simulink model "ARC_DTm"  (R2025b)
settings: Solver=FixedStepAuto  StartTime=0.0  StopTime=10080  FixedStep=1  RelTol=1e-3
PreLoadFcn:
  | %For Preload, set the working path
  | modelFolder = fileparts(which(bdroot));
  | addpath(genpath(modelFolder));
StartFcn:
  | tic
StopFcn:
  | fprintf("Sim Time: %.02f min", toc/60)
values from neighbouring files (symbols this model uses):
  batteryScenario = p.batteryScenario    [RUNSIM_ParameterSweep.m]    (also in _RUNSIM_ParameterSweep.m)
  Electricity_SalePriceModifier = 50/100    (= 0.5)    [RUNSIM_ParameterSweep.m]    (also in _RUNSIM_ParameterSweep.m)
  LUT = LUT_load.gamLUT    [RUNSIM_ParameterSweep.m]    (also in _RUNSIM_ParameterSweep.m)
  minimum_UF_system_flow = 5833    [RUNSIM_ParameterSweep.m]    (also in _RUNSIM_ParameterSweep.m)
  PROS1_recoveryrate = 61    [RUNSIM_ParameterSweep.m]    (also in _RUNSIM_ParameterSweep.m)
  PROS2_recoveryrate = 62    [RUNSIM_ParameterSweep.m]    (also in _RUNSIM_ParameterSweep.m)
  ROstabilization_time = p.ROstabilization_time    [RUNSIM_ParameterSweep.m]    (also in _RUNSIM_ParameterSweep.m)
  solarModifier = maximum_solar_generation / 300    [RUNSIM_ParameterSweep.m]    (also in _RUNSIM_ParameterSweep.m)
  TSRO_recoveryrate = 51    [RUNSIM_ParameterSweep.m]    (also in _RUNSIM_ParameterSweep.m)
  UF_RecoveryRate = 96    [RUNSIM_ParameterSweep.m]    (also in _RUNSIM_ParameterSweep.m)
undefined symbols (not defined in the file or in its folder): A_PROS1, A_PROS2, A_TSRO, B_PROS1, B_PROS2, B_TSRO, BW_Max_Time, BW_Max_Vol_gal, CEB_Max_Time, CEB_Max_Vol_gal, CIP_Max_Time, E, FF, h, L, w
libraries: simulink x40
(part 8 of 11)

== system ARC_DTm/Plant_LocalLoad_FMU/Battery System/Battery PID Solar Data1 ==
  note: M=2.5, kp=2.965, Ti=166.5, ki=0.0178
      |
      | M=1.5, kp=4.9, Ti=99.9, ki=0.049
      |
      | M=0.5, kp=14.8, Ti=33.3, ki=0.4
      |
      | M=0.1, kp=74.13, Ti=6.66, ki=11.13
      |
      | M=0.055 kp=134.79, Ti=3.663, ki=36.79
      |
      | M=0.01, kp=741.35, Ti=0.666, ki=1112.8
      |
      | M=0.001, kp=7413.5, Ti=0.0666, ki=111,313.81
      |
      | M=0.0001, kp=74135.09, Ti=0.00666, ki=11,113,394.89
  Setpoint : Inport
  feedback : Inport  Port=2
  Add : Sum
  BatteryCharge : Saturate  UpperLimit=0  LowerLimit=-1
  Constant : Constant  Value=0
  Dead Zone : DeadZone  LowerValue=-0.01  UpperValue=0.01
  Dead Zone1 : DeadZone  LowerValue=-0.025  UpperValue=0.025
  Gain7 : Gain  Gain=134.79
  Gain8 : Gain  Gain=36.79
  Manual Switch : ManualSwitch
  Proportional3 : Gain  SaturateOnIntegerOverflow=on  OutDataTypeStr=Inherit: Same as input  ParamDataTypeStr=Inherit: Same as input
  Scope : Scope  NumInputPorts=3
      settings: ActiveDisplayYMinimum=-113.50359317586926  ActiveDisplayYMaximum=90.190900765776917  DataLoggingVariableName=ScopeData4
  Scope1 : Scope
      settings: ActiveDisplayYMinimum=-1  ActiveDisplayYMaximum=1  DataLoggingVariableName=ScopeData8
  Scope2 : Scope  NumInputPorts=4
      settings: Title=Setpoint  ActiveDisplayYMinimum=-0.96522618550308326  ActiveDisplayYMaximum=1.0322332098634432  DataLoggingVariableName=ScopeData2
  Subtract : Sum  Inputs=+-
  Subtract1 : Sum  Inputs=+-
  Sum1 : Sum  Inputs=|+-
  Sum6 : Sum  Inputs=+-  InputSameDT=on  SaturateOnIntegerOverflow=on  OutDataTypeStr=Inherit: Same as first input
  Unit Delay : UnitDelay  SampleTime=-1  HasFrameUpgradeWarning=on
  Unit Delay1 : UnitDelay  SampleTime=-1  HasFrameUpgradeWarning=on
  open-loop steps : Subsystem
  Battery Disch : Outport
  wires:
  Manual Switch/1 -> Battery Disch/1
  open-loop steps/1(Out1) -> Manual Switch/2
  Setpoint/1 -> Scope2/1, Subtract1/1
  Proportional3/1 -> Subtract/2
  feedback/1 -> Scope2/2, Subtract1/2
  Sum1/1 -> Add/2, Unit Delay/1
  Subtract/1 -> Scope1/1, Sum1/1
  Unit Delay/1 -> Sum1/2
  Subtract1/1 -> Gain8/1, Gain7/1, Scope2/3
  BatteryCharge/1 -> Sum6/2, Scope2/4, Manual Switch/1, Scope/2
  Add/1 -> Scope/1, BatteryCharge/1, Sum6/1
  Gain7/1 -> Add/1
  Gain8/1 -> Subtract/1
  Sum6/1 -> Proportional3/1, Scope/3

== system ARC_DTm/Plant_LocalLoad_FMU/Battery System/Battery PID Solar Data2 ==
  note: M=2.5, kp=2.965, Ti=166.5, ki=0.0178
      |
      | M=1.5, kp=4.9, Ti=99.9, ki=0.049
      |
      | M=0.5, kp=14.8, Ti=33.3, ki=0.4
      |
      | M=0.1, kp=74.13, Ti=6.66, ki=11.13
      |
      | M=0.055 kp=134.79, Ti=3.663, ki=36.79
      |
      | M=0.01, kp=741.35, Ti=0.666, ki=1112.8
      |
      | M=0.001, kp=7413.5, Ti=0.0666, ki=111,313.81
      |
      | M=0.0001, kp=74135.09, Ti=0.00666, ki=11,113,394.89
  Setpoint : Inport
  feedback : Inport  Port=2
  Add : Sum
  BatteryCharge : Saturate  UpperLimit=1  LowerLimit=0
  Constant : Constant  Value=0
  Dead Zone : DeadZone  LowerValue=-0.01  UpperValue=0.01
  Dead Zone1 : DeadZone  LowerValue=-0.025  UpperValue=0.025
  Gain7 : Gain  Gain=134.79
  Gain8 : Gain  Gain=36.79
  Manual Switch : ManualSwitch
  Proportional3 : Gain  SaturateOnIntegerOverflow=on  OutDataTypeStr=Inherit: Same as input  ParamDataTypeStr=Inherit: Same as input
  Scope : Scope  NumInputPorts=3
      settings: ActiveDisplayYMinimum=-39.201768628012239  ActiveDisplayYMaximum=109.61089187015484  DataLoggingVariableName=ScopeData4
  Scope1 : Scope
      settings: ActiveDisplayYMinimum=-1  ActiveDisplayYMaximum=1  DataLoggingVariableName=ScopeData9
  Scope2 : Scope  NumInputPorts=4
      settings: Title=Setpoint  ActiveDisplayYMinimum=-0.96522618502196855  ActiveDisplayYMaximum=1.0322332055334107  DataLoggingVariableName=ScopeData2
  Scope3 : Scope  NumInputPorts=2
      settings: ActiveDisplayYMinimum=-0.25471317003362626  ActiveDisplayYMaximum=0.79251853030263664  DataLoggingVariableName=ScopeData2
  Subtract : Sum  Inputs=+-
  Subtract1 : Sum  Inputs=+-
  Sum1 : Sum  Inputs=|+-
  Sum6 : Sum  Inputs=+-  InputSameDT=on  SaturateOnIntegerOverflow=on  OutDataTypeStr=Inherit: Same as first input
  Unit Delay : UnitDelay  SampleTime=-1  HasFrameUpgradeWarning=on
  open-loop steps : Subsystem
  BatteryChargeDisch : Outport
  wires:
  Manual Switch/1 -> BatteryChargeDisch/1
  open-loop steps/1(Out1) -> Manual Switch/2
  Setpoint/1 -> Scope2/1, Subtract1/1
  Proportional3/1 -> Subtract/2
  feedback/1 -> Scope2/2, Subtract1/2
  Sum1/1 -> Add/2, Unit Delay/1
  Subtract/1 -> Scope1/1, Sum1/1
  Unit Delay/1 -> Sum1/2
  Subtract1/1 -> Scope3/2, Gain8/1, Gain7/1, Scope2/3, Scope3/1
  BatteryCharge/1 -> Scope2/4, Manual Switch/1, Sum6/2, Scope/2
  Add/1 -> Scope/1, Sum6/1, BatteryCharge/1
  Gain7/1 -> Add/1
  Gain8/1 -> Subtract/1
  Sum6/1 -> Proportional3/1, Scope/3

== system ARC_DTm/Plant_LocalLoad_FMU/Battery System/Battery PID Solar Data3 ==
  note: M=2.5, kp=2.965, Ti=166.5, ki=0.0178
      |
      | M=1.5, kp=4.9, Ti=99.9, ki=0.049
      |
      | M=0.5, kp=14.8, Ti=33.3, ki=0.4
      |
      | M=0.1, kp=74.13, Ti=6.66, ki=11.13
      |
      | M=0.055 kp=134.79, Ti=3.663, ki=36.79
      |
      | M=0.01, kp=741.35, Ti=0.666, ki=1112.8
      |
      | M=0.001, kp=7413.5, Ti=0.0666, ki=111,313.81
      |
      | M=0.0001, kp=74135.09, Ti=0.00666, ki=11,113,394.89
  Setpoint : Inport
  feedback : Inport  Port=2
  Add : Sum
  BatteryCharge : Saturate  UpperLimit=0  LowerLimit=-1
  Constant : Constant  Value=0
  Dead Zone : DeadZone  LowerValue=-0.01  UpperValue=0.01
  Dead Zone1 : DeadZone  LowerValue=-0.025  UpperValue=0.025
  Gain7 : Gain  Gain=134.79
  Gain8 : Gain  Gain=36.79
  Manual Switch : ManualSwitch
  Proportional3 : Gain  SaturateOnIntegerOverflow=on  OutDataTypeStr=Inherit: Same as input  ParamDataTypeStr=Inherit: Same as input
  Scope : Scope  NumInputPorts=3
      settings: ActiveDisplayYMinimum=-113.50359317586926  ActiveDisplayYMaximum=90.190900765776917  DataLoggingVariableName=ScopeData4
  Scope1 : Scope
      settings: ActiveDisplayYMinimum=-1  ActiveDisplayYMaximum=1  DataLoggingVariableName=ScopeData8
  Scope2 : Scope  NumInputPorts=4
      settings: Title=Setpoint  ActiveDisplayYMinimum=-0.96522618550308326  ActiveDisplayYMaximum=1.0322332098634432  DataLoggingVariableName=ScopeData2
  Subtract : Sum  Inputs=+-
  Subtract1 : Sum  Inputs=+-
  Sum1 : Sum  Inputs=|+-
  Sum6 : Sum  Inputs=+-  InputSameDT=on  SaturateOnIntegerOverflow=on  OutDataTypeStr=Inherit: Same as first input
  Unit Delay : UnitDelay  SampleTime=-1  HasFrameUpgradeWarning=on
  Unit Delay1 : UnitDelay  SampleTime=-1  HasFrameUpgradeWarning=on
  open-loop steps : Subsystem
  Battery Disch : Outport
  wires:
  Manual Switch/1 -> Battery Disch/1
  open-loop steps/1(Out1) -> Manual Switch/2
  Setpoint/1 -> Scope2/1, Subtract1/1
  Proportional3/1 -> Subtract/2
  feedback/1 -> Scope2/2, Subtract1/2
  Sum1/1 -> Add/2, Unit Delay/1
  Subtract/1 -> Scope1/1, Sum1/1
  Unit Delay/1 -> Sum1/2
  Subtract1/1 -> Gain8/1, Gain7/1, Scope2/3
  BatteryCharge/1 -> Sum6/2, Scope2/4, Manual Switch/1, Scope/2
  Add/1 -> Scope/1, BatteryCharge/1, Sum6/1
  Gain7/1 -> Add/1
  Gain8/1 -> Subtract/1
  Sum6/1 -> Proportional3/1, Scope/3

== system ARC_DTm/Plant_LocalLoad_FMU/Battery System/Excess Solar ==
  Solar In : Inport
  Local Load Demand : Inport  Port=2
  Action Port : ActionPort  ActionPortLabel=if(u1 == 1)
  Battery PID Solar Data : Subsystem  Commented=on
  Battery PID Solar Data1 : Subsystem  Commented=on
  Cast To Double : DataTypeConversion  OutDataTypeStr=double  SaturateOnIntegerOverflow=off  RndMeth=Floor
  Cast To Double1 : DataTypeConversion  OutDataTypeStr=double  SaturateOnIntegerOverflow=off  RndMeth=Floor
  Compare To Zero : simulink/Logic and Bit Operations/Compare To Zero  relop=>=  OutDataTypeStr=boolean
  Compare To Zero1 : simulink/Logic and Bit Operations/Compare To Zero  relop=<  OutDataTypeStr=boolean
  From1 : From  Commented=on  GotoTag=SOC
  From2 : From  Commented=on  GotoTag=SOC
  Gain : Gain  Commented=on  Gain=-1
  Goto : Goto  Commented=on  GotoTag=SOC
  Scope : Scope  Commented=on  NumInputPorts=2
      settings: ActiveDisplayYMinimum=-1.0125  ActiveDisplayYMaximum=0.11249999999999998  DataLoggingVariableName=ScopeData27
  Scope1 : Scope  Commented=on  NumInputPorts=2
      settings: ActiveDisplayYMinimum=-0.96522618502196855  ActiveDisplayYMaximum=1.0322332055334107  DataLoggingVariableName=ScopeData37
  "Setpoint PID Solar+Battery " : Subsystem  Commented=on
  Sum : Sum  Inputs=|+-
  Unit Delay1 : UnitDelay  Commented=on  SampleTime=-1  HasFrameUpgradeWarning=on
  Unit Delay2 : UnitDelay  Commented=on  SampleTime=-1  HasFrameUpgradeWarning=on
  Battery Charge Command : Outport
  Battery Discharge Command : Outport  Port=2
  wires:
  Gain/1 -> Scope/2
  Unit Delay2/1 -> Battery PID Solar Data1/2(feedback)
  "Setpoint PID Solar+Battery "/2(Setpoint BattDischarge) -> Scope/1, Battery PID Solar Data1/1(Setpoint)
  "Setpoint PID Solar+Battery "/1(Setpoint BattCharge) -> Scope1/1, Battery PID Solar Data/1(Setpoint)
  From1/1 -> Unit Delay1/1
  Battery PID Solar Data1/1(Battery Disch) -> Gain/1
  From2/1 -> Unit Delay2/1
  Unit Delay1/1 -> Battery PID Solar Data/2(feedback)
  Battery PID Solar Data/1(BatteryChargeDisch) -> Scope1/2
  Solar In/1 -> Sum/1
  Local Load Demand/1 -> Sum/2
  Sum/1 -> Compare To Zero1/1, Compare To Zero/1
  Compare To Zero/1 -> Cast To Double1/1
  Compare To Zero1/1 -> Cast To Double/1
  Cast To Double/1 -> Battery Discharge Command/1
  Cast To Double1/1 -> Battery Charge Command/1

== system ARC_DTm/Plant_LocalLoad_FMU/Battery System/NoBattery ==
  Action Port : ActionPort  ActionPortLabel=else
  No Charge : Constant  Value=0
  Battery Charge Request : Outport
  Battery Discharge Request : Outport  Port=2
  wires:
  No Charge/1 -> Battery Discharge Request/1, Battery Charge Request/1

== system ARC_DTm/Plant_LocalLoad_FMU/Battery System/Setpoint PID Solar+Battery  ==
  Solar Power : Inport
  Local Load Demand : Inport  Port=2
  Divide : Product  Inputs=*/
  Rate Limiter1 : RateLimiter  RisingSlewLimit=0.00000607  FallingSlewLimit=-0.00000607  SampleTimeMode=inherited
  Rate Limiter2 : RateLimiter  RisingSlewLimit=0.00000607  FallingSlewLimit=-0.00000607  SampleTimeMode=inherited
  Saturation1 : Saturate  UpperLimit=0.9  LowerLimit=-0.9
  Saturation4 : Saturate  UpperLimit=0.9  LowerLimit=-0.9
  Scaling factor Solar Data to 1 MW Battery : Constant  Value=10000
  Scope7 : Scope  NumInputPorts=3
      settings: Title=Battery Charge/Discharge SOC Output  ActiveDisplayYMinimum=-0.95011803109224124  ActiveDisplayYMaximum=0.10556867012136011
  Subtract2 : Sum  Inputs=+-
  Transfer Fcn3 : TransferFcn  Denominator=[300 1]
  Setpoint BattCharge : Outport
  Setpoint BattDischarge : Outport  Port=2
  wires:
  Subtract2/1 -> Scope7/1, Transfer Fcn3/1
  Transfer Fcn3/1 -> Divide/1
  Local Load Demand/1 -> Subtract2/2
  Solar Power/1 -> Subtract2/1
  Divide/1 -> Saturation1/1, Saturation4/1
  Saturation4/1 -> Setpoint BattCharge/1, Scope7/2
  Saturation1/1 -> Scope7/3, Setpoint BattDischarge/1
  Scaling factor Solar Data to 1 MW Battery/1 -> Divide/2

== system ARC_DTm/Product Water Tank/Tank Storage/Manage Overflows ==
  Timer : Inport
  <Flow Rate (FLOW)> : Inport  Port=2
  <Permeate Flow (FLOW)> : Inport  Port=3
  Pump Flow (FLOW) : Inport  Port=4
  If : If  IfExpression=u1 >= 1  ElseIfExpressions=u1<= -1
  If Action Subsystem : Subsystem  TreatAsAtomicUnit=on
  If Action Subsystem1 : Subsystem  TreatAsAtomicUnit=on
  Merge : Merge  Inputs=3
  Merge1 : Merge  Inputs=3
  Merge2 : Merge  Inputs=3
  Pump Flow Reduction : Subsystem  TreatAsAtomicUnit=on
  Reduce to Zero : MATLAB Function  TreatAsAtomicUnit=on
  Scope : Scope
      settings: ActiveDisplayYMinimum=-18.75  ActiveDisplayYMaximum=18.75  DataLoggingVariableName=ScopeData2
  Well Flow Rate (FLOW) : Outport
  RO Perm Flow Rate (FLOW) : Outport  Port=2
  Pump Flow Rate (FLOW) : Outport  Port=3
  TimerOut : Outport  Port=4
  wires:
  Timer/1 -> Reduce to Zero/1(u), Scope/1, If/1
  If/1 -> If Action Subsystem/Action
  <Flow Rate (FLOW)>/1 -> Pump Flow Reduction/1(<Flow Rate (FLOW)>), If Action Subsystem/1(<Flow Rate (FLOW)>), If Action Subsystem1/1(<Flow Rate (FLOW)>)
  <Permeate Flow (FLOW)>/1 -> Pump Flow Reduction/2(<PermeateFlow (FLOW)>), If Action Subsystem/2(<Permeate Flow (FLOW)>), If Action Subsystem1/2(<Permeate Flow (FLOW)>)
  Pump Flow (FLOW)/1 -> If Action Subsystem/3(Pump Flow (FLOW)), If Action Subsystem1/3(<Pump Flow (FLOW)>)
  If Action Subsystem/1(Raw Water Flow Rate (FLOW)) -> Merge/1
  If/3 -> If Action Subsystem1/Action
  If Action Subsystem1/1(Well Flow Rate (FLOW)) -> Merge/2
  Merge/1 -> Well Flow Rate (FLOW)/1
  If Action Subsystem/2(RO Permeate Flow Rate (FLOW)) -> Merge1/1
  If Action Subsystem1/2(RO Perm Flow Rate (FLOW)) -> Merge1/2
  Merge1/1 -> RO Perm Flow Rate (FLOW)/1
  Pump Flow Reduction/3(Pump Flow (FLOW)) -> Merge2/3
  Merge2/1 -> Pump Flow Rate (FLOW)/1
  If/2 -> Pump Flow Reduction/Action
  If Action Subsystem1/3(Pump Flow (FLOW)) -> Merge2/2
  If Action Subsystem/3(Pump Flow Rate (FLOW)) -> Merge2/1
  Pump Flow Reduction/2(Permeate Flow Rate (FLOW)) -> Merge1/3
  Pump Flow Reduction/1(Well Flow Rate (FLOW)) -> Merge/3
  Reduce to Zero/1(y) -> TimerOut/1

== system ARC_DTm/Product Water Tank/Tank Storage/VolumeConditions ==
  note: Volume Overflow
  Stored Volume (VOL) : Inport
  Tank Volume (VOL) : Inport  Port=2
  Timer : Inport  Port=3
  If : If  NumInputs=3  IfExpression=u1 >= u2  ElseIfExpressions=u1 <= u3, u3 < u1 < u2  ShowElse=off
  MaximumOperationalVolume : Gain  Gain=volMax
  Merge : Merge  Inputs=3
  MinimumOperationalVolume : Gain  Gain=volMin
  Scope : Scope
      settings: ActiveDisplayYMinimum=-1  ActiveDisplayYMaximum=1  DataLoggingVariableName=ScopeData3
  Tank Above Operating Range : Subsystem  TreatAsAtomicUnit=on
  Tank Below Operating Range : Subsystem  TreatAsAtomicUnit=on
  Tank in Operating Range : Subsystem  TreatAsAtomicUnit=on
  Cooldown Timer : Outport
  wires:
  Tank in Operating Range/1(y) -> Merge/2
  Stored Volume (VOL)/1 -> If/1
  If/1 -> Tank Above Operating Range/Action
  Tank Above Operating Range/1(Out1) -> Merge/1
  Merge/1 -> Scope/1, Cooldown Timer/1
  If/2 -> Tank in Operating Range/Action
  If/3 -> Tank Below Operating Range/Action
  Tank Below Operating Range/1(Out1) -> Merge/3
  Tank Volume (VOL)/1 -> MinimumOperationalVolume/1, MaximumOperationalVolume/1
  MaximumOperationalVolume/1 -> If/2
  MinimumOperationalVolume/1 -> If/3
  Timer/1 -> Tank in Operating Range/1(Timer)

== system ARC_DTm/UF Maintenance Coordinator/arhive/UF_Operation State_1 ==
  UF1_MaintenanceStartSignal : Inport
  UF1_BeginStandby : Inport  Port=2
  UF1_BeginStartup : Inport  Port=3
  Bus Creator : BusCreator  Inputs=2
  Bus Selector : BusSelector  OutputSignals=UF_ShutdownCmd_1
  Bus Selector1 : BusSelector  OutputSignals=UF_MaintCmd_1
  Bus Selector2 : BusSelector  OutputSignals=UF_StartupCmd_1
  Delay Reset Signal : Memory
  Delay Startup : Memory
  UF1_Maintenance State : Stateflow chart  TreatAsAtomicUnit=on
  tag scope: UF1_MaintenanceRequest=global, UF1_MaintenanceState=global, UF1_OperatingState=global, UF1_StartupRequest=global
  wires:
  UF1_Maintenance State/1(unit_in_maint_queue) -> [UF1_MaintenanceRequest]  "UF1_MaintenanceRequestQueue"
  Bus Creator/1 -> [UF1_MaintenanceState]
  Delay Startup/1 -> [UF1_OperatingState], Bus Creator/1  "UF1_OperationsState"
  UF1_Maintenance State/4(maintenance_completion_indicator) -> Delay Reset Signal/1  "UF1_MaintenanceCompletionSignal"
  [UF1_Maintenance_Request] -> UF1_Maintenance State/2(maint_req)
  Delay Reset Signal/1 -> Bus Creator/2  "UF1_MaintenanceCompletionSignal"
  UF1_Maintenance State/3(unit_in_operation) -> Delay Startup/1  "UF1_OperationsState"
  UF1_Maintenance State/2(unit_in_startup_queue) -> [UF1_StartupRequest]  "UF1_StartupRequestQueue"
  UF1_BeginStandby/1 -> Bus Selector/1  "UF1_BeginStandby"
  Bus Selector/1 -> UF1_Maintenance State/3(standby_cmd)  "<UF_ShutdownCmd_1>"
  UF1_MaintenanceStartSignal/1 -> Bus Selector1/1  "UF1_MaintenanceStartSignal"
  Bus Selector1/1 -> UF1_Maintenance State/1(maint_cmd)  "<UF_MaintCmd_1>"
  UF1_BeginStartup/1 -> Bus Selector2/1  "UF1_BeginStartup"
  Bus Selector2/1 -> UF1_Maintenance State/4(startup_cmd)  "<UF_StartupCmd_1>"

== system ARC_DTm/UF Maintenance Coordinator/arhive/UF_Operation State_10 ==
  UF10_MaintenanceStartSignal : Inport
  UF10_BeginStandby : Inport  Port=2
  UF10_BeginStartup : Inport  Port=3
  Bus Creator : BusCreator  Inputs=2
  Bus Selector : BusSelector  OutputSignals=UF_ShutdownCmd_10
  Bus Selector10 : BusSelector  OutputSignals=UF_MaintCmd_10
  Bus Selector2 : BusSelector  OutputSignals=UF_StartupCmd_10
  Delay Reset Signal : Memory
  Delay Startup : Memory
  UF10_Maintenance State : Stateflow chart  TreatAsAtomicUnit=on
  tag scope: UF10_MaintenanceRequest=global, UF10_MaintenanceState=global, UF10_OperatingState=global, UF10_StartupRequest=global
  wires:
  UF10_Maintenance State/1(unit_in_maint_queue) -> [UF10_MaintenanceRequest]  "UF10_MaintenanceRequestQueue"
  Bus Creator/1 -> [UF10_MaintenanceState]
  Delay Startup/1 -> [UF10_OperatingState], Bus Creator/1  "UF10_OperationsState"
  UF10_Maintenance State/4(maintenance_completion_indicator) -> Delay Reset Signal/1  "UF10_MaintenanceCompletionSignal"
  [UF10_Maintenance_Request] -> UF10_Maintenance State/2(maint_req)
  Delay Reset Signal/1 -> Bus Creator/2  "UF10_MaintenanceCompletionSignal"
  UF10_Maintenance State/3(unit_in_operation) -> Delay Startup/1  "UF10_OperationsState"
  UF10_Maintenance State/2(unit_in_startup_queue) -> [UF10_StartupRequest]  "UF10_StartupRequestQueue"
  UF10_BeginStandby/1 -> Bus Selector/1  "UF10_BeginStandby"
  Bus Selector/1 -> UF10_Maintenance State/3(standby_cmd)  "<UF_ShutdownCmd_10>"
  UF10_MaintenanceStartSignal/1 -> Bus Selector10/1  "UF10_MaintenanceStartSignal"
  Bus Selector10/1 -> UF10_Maintenance State/1(maint_cmd)  "<UF_MaintCmd_10>"
  UF10_BeginStartup/1 -> Bus Selector2/1  "UF10_BeginStartup"
  Bus Selector2/1 -> UF10_Maintenance State/4(startup_cmd)  "<UF_StartupCmd_10>"

== system ARC_DTm/UF Maintenance Coordinator/arhive/UF_Operation State_2 ==
  UF2_MaintenanceStartSignal : Inport
  UF2_BeginStandby : Inport  Port=2
  UF2_BeginStartup : Inport  Port=3
  Bus Creator : BusCreator  Inputs=2
  Bus Selector : BusSelector  OutputSignals=UF_ShutdownCmd_2
  Bus Selector1 : BusSelector  OutputSignals=UF_MaintCmd_2
  Bus Selector2 : BusSelector  OutputSignals=UF_StartupCmd_2
  Delay Reset Signal : Memory
  Delay Startup : Memory
  UF2_Maintenance State : Stateflow chart  TreatAsAtomicUnit=on
  tag scope: UF2_MaintenanceRequest=global, UF2_MaintenanceState=global, UF2_OperatingState=global, UF2_StartupRequest=global
  wires:
  UF2_Maintenance State/1(unit_in_maint_queue) -> [UF2_MaintenanceRequest]  "UF2_MaintenanceRequestQueue"
  Bus Creator/1 -> [UF2_MaintenanceState]
  UF2_Maintenance State/4(maintenance_completion_indicator) -> Delay Reset Signal/1  "UF2_MaintenanceCompletionSignal"
  [UF2_Maintenance_Request] -> UF2_Maintenance State/2(maint_req)
  Delay Reset Signal/1 -> Bus Creator/2  "UF2_MaintenanceCompletionSignal"
  UF2_Maintenance State/3(unit_in_operation) -> Delay Startup/1  "UF2_OperationsState"
  UF2_Maintenance State/2(unit_in_startup_queue) -> [UF2_StartupRequest]  "UF2_StartupRequestQueue"
  UF2_BeginStandby/1 -> Bus Selector/1  "UF2_BeginStandby"
  Bus Selector/1 -> UF2_Maintenance State/3(standby_cmd)  "<UF_ShutdownCmd_2>"
  UF2_MaintenanceStartSignal/1 -> Bus Selector1/1  "UF2_MaintenanceStartSignal"
  Bus Selector1/1 -> UF2_Maintenance State/1(maint_cmd)  "<UF_MaintCmd_2>"
  UF2_BeginStartup/1 -> Bus Selector2/1  "UF2_BeginStartup"
  Bus Selector2/1 -> UF2_Maintenance State/4(startup_cmd)  "<UF_StartupCmd_2>"
  Delay Startup/1 -> [UF2_OperatingState], Bus Creator/1  "UF2_OperationsState"

== system ARC_DTm/UF Maintenance Coordinator/arhive/UF_Operation State_3 ==
  UF3_MaintenanceStartSignal : Inport
  UF3_BeginStandby : Inport  Port=2
  UF3_BeginStartup : Inport  Port=3
  Bus Creator : BusCreator  Inputs=2
  Bus Selector : BusSelector  OutputSignals=UF_ShutdownCmd_3
  Bus Selector2 : BusSelector  OutputSignals=UF_StartupCmd_3
  Bus Selector3 : BusSelector  OutputSignals=UF_MaintCmd_3
  Delay Reset Signal : Memory
  Delay Startup : Memory
  UF3_Maintenance State : Stateflow chart  TreatAsAtomicUnit=on
  tag scope: UF3_MaintenanceRequest=global, UF3_MaintenanceState=global, UF3_OperatingState=global, UF3_StartupRequest=global
  wires:
  UF3_Maintenance State/1(unit_in_maint_queue) -> [UF3_MaintenanceRequest]  "UF3_MaintenanceRequestQueue"
  Bus Creator/1 -> [UF3_MaintenanceState]
  Delay Startup/1 -> [UF3_OperatingState], Bus Creator/1  "UF3_OperationsState"
  UF3_Maintenance State/4(maintenance_completion_indicator) -> Delay Reset Signal/1  "UF3_MaintenanceCompletionSignal"
  [UF3_Maintenance_Request] -> UF3_Maintenance State/2(maint_req)
  Delay Reset Signal/1 -> Bus Creator/2  "UF3_MaintenanceCompletionSignal"
  UF3_Maintenance State/3(unit_in_operation) -> Delay Startup/1  "UF3_OperationsState"
  UF3_Maintenance State/2(unit_in_startup_queue) -> [UF3_StartupRequest]  "UF3_StartupRequestQueue"
  UF3_BeginStandby/1 -> Bus Selector/1  "UF3_BeginStandby"
  Bus Selector/1 -> UF3_Maintenance State/3(standby_cmd)  "<UF_ShutdownCmd_3>"
  UF3_MaintenanceStartSignal/1 -> Bus Selector3/1  "UF3_MaintenanceStartSignal"
  Bus Selector3/1 -> UF3_Maintenance State/1(maint_cmd)  "<UF_MaintCmd_3>"
  UF3_BeginStartup/1 -> Bus Selector2/1  "UF3_BeginStartup"
  Bus Selector2/1 -> UF3_Maintenance State/4(startup_cmd)  "<UF_StartupCmd_3>"

== system ARC_DTm/UF Maintenance Coordinator/arhive/UF_Operation State_4 ==
  UF4_MaintenanceStartSignal : Inport
  UF4_BeginStandby : Inport  Port=2
  UF4_BeginStartup : Inport  Port=3
  Bus Creator : BusCreator  Inputs=2
  Bus Selector : BusSelector  OutputSignals=UF_ShutdownCmd_4
  Bus Selector2 : BusSelector  OutputSignals=UF_StartupCmd_4
  Bus Selector4 : BusSelector  OutputSignals=UF_MaintCmd_4
  Delay Reset Signal : Memory
  Delay Startup : Memory
  UF4_Maintenance State : Stateflow chart  TreatAsAtomicUnit=on
  tag scope: UF4_MaintenanceRequest=global, UF4_MaintenanceState=global, UF4_OperatingState=global, UF4_StartupRequest=global
  wires:
  UF4_Maintenance State/1(unit_in_maint_queue) -> [UF4_MaintenanceRequest]  "UF4_MaintenanceRequestQueue"
  Bus Creator/1 -> [UF4_MaintenanceState]
  Delay Startup/1 -> [UF4_OperatingState], Bus Creator/1  "UF4_OperationsState"
  UF4_Maintenance State/4(maintenance_completion_indicator) -> Delay Reset Signal/1  "UF4_MaintenanceCompletionSignal"
  [UF4_Maintenance_Request] -> UF4_Maintenance State/2(maint_req)
  Delay Reset Signal/1 -> Bus Creator/2  "UF4_MaintenanceCompletionSignal"
  UF4_Maintenance State/3(unit_in_operation) -> Delay Startup/1  "UF4_OperationsState"
  UF4_Maintenance State/2(unit_in_startup_queue) -> [UF4_StartupRequest]  "UF4_StartupRequestQueue"
  UF4_BeginStandby/1 -> Bus Selector/1  "UF4_BeginStandby"
  Bus Selector/1 -> UF4_Maintenance State/3(standby_cmd)  "<UF_ShutdownCmd_4>"
  UF4_MaintenanceStartSignal/1 -> Bus Selector4/1  "UF4_MaintenanceStartSignal"
  Bus Selector4/1 -> UF4_Maintenance State/1(maint_cmd)  "<UF_MaintCmd_4>"
  UF4_BeginStartup/1 -> Bus Selector2/1  "UF4_BeginStartup"
  Bus Selector2/1 -> UF4_Maintenance State/4(startup_cmd)  "<UF_StartupCmd_4>"

== system ARC_DTm/UF Maintenance Coordinator/arhive/UF_Operation State_5 ==
  UF5_MaintenanceStartSignal : Inport
  UF5_BeginStandby : Inport  Port=2
  UF5_BeginStartup : Inport  Port=3
  Bus Creator : BusCreator  Inputs=2
  Bus Selector : BusSelector  OutputSignals=UF_ShutdownCmd_5
  Bus Selector2 : BusSelector  OutputSignals=UF_StartupCmd_5
  Bus Selector5 : BusSelector  OutputSignals=UF_MaintCmd_5
  Delay Reset Signal : Memory
  Delay Startup : Memory
  UF5_Maintenance State : Stateflow chart  TreatAsAtomicUnit=on
  tag scope: UF5_MaintenanceRequest=global, UF5_MaintenanceState=global, UF5_OperatingState=global, UF5_StartupRequest=global
  wires:
  UF5_Maintenance State/1(unit_in_maint_queue) -> [UF5_MaintenanceRequest]  "UF5_MaintenanceRequestQueue"
  Bus Creator/1 -> [UF5_MaintenanceState]
  Delay Startup/1 -> [UF5_OperatingState], Bus Creator/1  "UF5_OperationsState"
  UF5_Maintenance State/4(maintenance_completion_indicator) -> Delay Reset Signal/1  "UF5_MaintenanceCompletionSignal"
  [UF5_Maintenance_Request] -> UF5_Maintenance State/2(maint_req)
  Delay Reset Signal/1 -> Bus Creator/2  "UF5_MaintenanceCompletionSignal"
  UF5_Maintenance State/3(unit_in_operation) -> Delay Startup/1  "UF5_OperationsState"
  UF5_Maintenance State/2(unit_in_startup_queue) -> [UF5_StartupRequest]  "UF5_StartupRequestQueue"
  UF5_BeginStandby/1 -> Bus Selector/1  "UF5_BeginStandby"
  Bus Selector/1 -> UF5_Maintenance State/3(standby_cmd)  "<UF_ShutdownCmd_5>"
  UF5_MaintenanceStartSignal/1 -> Bus Selector5/1  "UF5_MaintenanceStartSignal"
  Bus Selector5/1 -> UF5_Maintenance State/1(maint_cmd)  "<UF_MaintCmd_5>"
  UF5_BeginStartup/1 -> Bus Selector2/1  "UF5_BeginStartup"
  Bus Selector2/1 -> UF5_Maintenance State/4(startup_cmd)  "<UF_StartupCmd_5>"

== system ARC_DTm/UF Maintenance Coordinator/arhive/UF_Operation State_6 ==
  UF6_MaintenanceStartSignal : Inport
  UF6_BeginStandby : Inport  Port=2
  UF6_BeginStartup : Inport  Port=3
  Bus Creator : BusCreator  Inputs=2
  Bus Selector : BusSelector  OutputSignals=UF_ShutdownCmd_6
  Bus Selector2 : BusSelector  OutputSignals=UF_StartupCmd_6
  Bus Selector6 : BusSelector  OutputSignals=UF_MaintCmd_6
  Delay Reset Signal : Memory
  Delay Startup : Memory
  UF6_Maintenance State : Stateflow chart  TreatAsAtomicUnit=on
  tag scope: UF6_MaintenanceRequest=global, UF6_MaintenanceState=global, UF6_OperatingState=global, UF6_StartupRequest=global
  wires:
  UF6_Maintenance State/1(unit_in_maint_queue) -> [UF6_MaintenanceRequest]  "UF6_MaintenanceRequestQueue"
  Bus Creator/1 -> [UF6_MaintenanceState]
  Delay Startup/1 -> [UF6_OperatingState], Bus Creator/1  "UF6_OperationsState"
  UF6_Maintenance State/4(maintenance_completion_indicator) -> Delay Reset Signal/1  "UF6_MaintenanceCompletionSignal"
  [UF6_Maintenance_Request] -> UF6_Maintenance State/2(maint_req)
  Delay Reset Signal/1 -> Bus Creator/2  "UF6_MaintenanceCompletionSignal"
  UF6_Maintenance State/3(unit_in_operation) -> Delay Startup/1  "UF6_OperationsState"
  UF6_Maintenance State/2(unit_in_startup_queue) -> [UF6_StartupRequest]  "UF6_StartupRequestQueue"
  UF6_BeginStandby/1 -> Bus Selector/1  "UF6_BeginStandby"
  Bus Selector/1 -> UF6_Maintenance State/3(standby_cmd)  "<UF_ShutdownCmd_6>"
  UF6_MaintenanceStartSignal/1 -> Bus Selector6/1  "UF6_MaintenanceStartSignal"
  Bus Selector6/1 -> UF6_Maintenance State/1(maint_cmd)  "<UF_MaintCmd_6>"
  UF6_BeginStartup/1 -> Bus Selector2/1  "UF6_BeginStartup"
  Bus Selector2/1 -> UF6_Maintenance State/4(startup_cmd)  "<UF_StartupCmd_6>"

== system ARC_DTm/UF Maintenance Coordinator/arhive/UF_Operation State_7 ==
  UF7_MaintenanceStartSignal : Inport
  UF7_BeginStandby : Inport  Port=2
  UF7_BeginStartup : Inport  Port=3
  Bus Creator : BusCreator  Inputs=2
  Bus Selector : BusSelector  OutputSignals=UF_ShutdownCmd_7
  Bus Selector2 : BusSelector  OutputSignals=UF_StartupCmd_7
  Bus Selector7 : BusSelector  OutputSignals=UF_MaintCmd_7
  Delay Reset Signal : Memory
  Delay Startup : Memory
  UF7_Maintenance State : Stateflow chart  TreatAsAtomicUnit=on
  tag scope: UF7_MaintenanceRequest=global, UF7_MaintenanceState=global, UF7_OperatingState=global, UF7_StartupRequest=global
  wires:
  UF7_Maintenance State/1(unit_in_maint_queue) -> [UF7_MaintenanceRequest]  "UF7_MaintenanceRequestQueue"
  Bus Creator/1 -> [UF7_MaintenanceState]
  Delay Startup/1 -> [UF7_OperatingState], Bus Creator/1  "UF7_OperationsState"
  UF7_Maintenance State/4(maintenance_completion_indicator) -> Delay Reset Signal/1  "UF7_MaintenanceCompletionSignal"
  [UF7_Maintenance_Request] -> UF7_Maintenance State/2(maint_req)
  Delay Reset Signal/1 -> Bus Creator/2  "UF7_MaintenanceCompletionSignal"
  UF7_Maintenance State/3(unit_in_operation) -> Delay Startup/1  "UF7_OperationsState"
  UF7_Maintenance State/2(unit_in_startup_queue) -> [UF7_StartupRequest]  "UF7_StartupRequestQueue"
  UF7_BeginStandby/1 -> Bus Selector/1  "UF7_BeginStandby"
  Bus Selector/1 -> UF7_Maintenance State/3(standby_cmd)  "<UF_ShutdownCmd_7>"
  UF7_MaintenanceStartSignal/1 -> Bus Selector7/1  "UF7_MaintenanceStartSignal"
  Bus Selector7/1 -> UF7_Maintenance State/1(maint_cmd)  "<UF_MaintCmd_7>"
  UF7_BeginStartup/1 -> Bus Selector2/1  "UF7_BeginStartup"
  Bus Selector2/1 -> UF7_Maintenance State/4(startup_cmd)  "<UF_StartupCmd_7>"

== system ARC_DTm/UF Maintenance Coordinator/arhive/UF_Operation State_8 ==
  UF8_MaintenanceStartSignal : Inport
  UF8_BeginStandby : Inport  Port=2
  UF8_BeginStartup : Inport  Port=3
  Bus Creator : BusCreator  Inputs=2
  Bus Selector : BusSelector  OutputSignals=UF_ShutdownCmd_8
  Bus Selector2 : BusSelector  OutputSignals=UF_StartupCmd_8
  Bus Selector8 : BusSelector  OutputSignals=UF_MaintCmd_8
  Delay Reset Signal : Memory
  Delay Startup : Memory
  UF8_Maintenance State : Stateflow chart  TreatAsAtomicUnit=on
  tag scope: UF8_MaintenanceRequest=global, UF8_MaintenanceState=global, UF8_OperatingState=global, UF8_StartupRequest=global
  wires:
  UF8_Maintenance State/1(unit_in_maint_queue) -> [UF8_MaintenanceRequest]  "UF8_MaintenanceRequestQueue"
  Bus Creator/1 -> [UF8_MaintenanceState]
  UF8_Maintenance State/4(maintenance_completion_indicator) -> Delay Reset Signal/1  "UF8_MaintenanceCompletionSignal"
  [UF8_Maintenance_Request] -> UF8_Maintenance State/2(maint_req)
  Delay Reset Signal/1 -> Bus Creator/2  "UF8_MaintenanceCompletionSignal"
  UF8_Maintenance State/3(unit_in_operation) -> Delay Startup/1  "UF8_OperationsState"
  UF8_Maintenance State/2(unit_in_startup_queue) -> [UF8_StartupRequest]  "UF8_StartupRequestQueue"
  UF8_BeginStandby/1 -> Bus Selector/1  "UF8_BeginStandby"
  Bus Selector/1 -> UF8_Maintenance State/3(standby_cmd)  "<UF_ShutdownCmd_8>"
  UF8_MaintenanceStartSignal/1 -> Bus Selector8/1  "UF8_MaintenanceStartSignal"
  Bus Selector8/1 -> UF8_Maintenance State/1(maint_cmd)  "<UF_MaintCmd_8>"
  UF8_BeginStartup/1 -> Bus Selector2/1  "UF8_BeginStartup"
  Bus Selector2/1 -> UF8_Maintenance State/4(startup_cmd)  "<UF_StartupCmd_8>"
  Delay Startup/1 -> [UF8_OperatingState], Bus Creator/1  "UF8_OperationsState"

== system ARC_DTm/UF Maintenance Coordinator/arhive/UF_Operation State_9 ==
  UF9_MaintenanceStartSignal : Inport
  UF9_BeginStandby : Inport  Port=2
  UF9_BeginStartup : Inport  Port=3
  Bus Creator : BusCreator  Inputs=2
  Bus Selector : BusSelector  OutputSignals=UF_ShutdownCmd_9
  Bus Selector2 : BusSelector  OutputSignals=UF_StartupCmd_9
  Bus Selector9 : BusSelector  OutputSignals=UF_MaintCmd_9
  Delay Reset Signal : Memory
  Delay Startup : Memory
  UF9_Maintenance State : Stateflow chart  TreatAsAtomicUnit=on
  tag scope: UF9_MaintenanceRequest=global, UF9_MaintenanceState=global, UF9_OperatingState=global, UF9_StartupRequest=global
  wires:
  UF9_Maintenance State/1(unit_in_maint_queue) -> [UF9_MaintenanceRequest]  "UF9_MaintenanceRequestQueue"
  Bus Creator/1 -> [UF9_MaintenanceState]
  Delay Startup/1 -> [UF9_OperatingState], Bus Creator/1  "UF9_OperationsState"
  UF9_Maintenance State/4(maintenance_completion_indicator) -> Delay Reset Signal/1  "UF9_MaintenanceCompletionSignal"
  [UF9_Maintenance_Request] -> UF9_Maintenance State/2(maint_req)
  Delay Reset Signal/1 -> Bus Creator/2  "UF9_MaintenanceCompletionSignal"
  UF9_Maintenance State/3(unit_in_operation) -> Delay Startup/1  "UF9_OperationsState"
  UF9_Maintenance State/2(unit_in_startup_queue) -> [UF9_StartupRequest]  "UF9_StartupRequestQueue"
  UF9_BeginStandby/1 -> Bus Selector/1  "UF9_BeginStandby"
  Bus Selector/1 -> UF9_Maintenance State/3(standby_cmd)  "<UF_ShutdownCmd_9>"
  UF9_MaintenanceStartSignal/1 -> Bus Selector9/1  "UF9_MaintenanceStartSignal"
  Bus Selector9/1 -> UF9_Maintenance State/1(maint_cmd)  "<UF_MaintCmd_9>"
  UF9_BeginStartup/1 -> Bus Selector2/1  "UF9_BeginStartup"
  Bus Selector2/1 -> UF9_Maintenance State/4(startup_cmd)  "<UF_StartupCmd_9>"

== system ARC_DTm/Plant_LocalLoad_FMU/Battery System/Battery PID Solar Data/open-loop steps ==
  Scope : Scope
      settings: ActiveDisplayYMinimum=-1.125  ActiveDisplayYMaximum=0.125
  Step : Step  Time=10000  SampleTime=0
  Step1 : Step  Time=46500  After=-1  SampleTime=0
  Step2 : Step  Time=60000  After=-1  SampleTime=0
  Step3 : Step  Time=90000  SampleTime=0
  Subtract : Sum
  Subtract1 : Sum
  Subtract2 : Sum
  Out1 : Outport
  wires:
  Step/1 -> Subtract/1
  Step1/1 -> Subtract/2
  Step2/1 -> Subtract1/1
  Subtract/1 -> Subtract2/1
  Subtract1/1 -> Subtract2/2, Scope/1
  Subtract2/1 -> Out1/1
  Step3/1 -> Subtract1/2

== system ARC_DTm/Plant_LocalLoad_FMU/Battery System/Battery PID Solar Data1/open-loop steps ==
  Scope : Scope
      settings: ActiveDisplayYMinimum=-1.125  ActiveDisplayYMaximum=0.125
  Step : Step  Time=10000  SampleTime=0
  Step1 : Step  Time=46500  After=-1  SampleTime=0
  Step2 : Step  Time=60000  After=-1  SampleTime=0
  Step3 : Step  Time=90000  SampleTime=0
  Subtract : Sum
  Subtract1 : Sum
  Subtract2 : Sum
  Out1 : Outport
  wires:
  Step/1 -> Subtract/1
  Step1/1 -> Subtract/2
  Step2/1 -> Subtract1/1
  Subtract/1 -> Subtract2/1
  Subtract1/1 -> Subtract2/2, Scope/1
  Subtract2/1 -> Out1/1
  Step3/1 -> Subtract1/2

== system ARC_DTm/Plant_LocalLoad_FMU/Battery System/Battery PID Solar Data2/open-loop steps ==
  Scope : Scope
      settings: ActiveDisplayYMinimum=-1.125  ActiveDisplayYMaximum=0.125
  Step : Step  Time=10000  SampleTime=0
  Step1 : Step  Time=46500  After=-1  SampleTime=0
  Step2 : Step  Time=60000  After=-1  SampleTime=0
  Step3 : Step  Time=90000  SampleTime=0
  Subtract : Sum
  Subtract1 : Sum
  Subtract2 : Sum
  Out1 : Outport
  wires:
  Step/1 -> Subtract/1
  Step1/1 -> Subtract/2
  Step2/1 -> Subtract1/1
  Subtract/1 -> Subtract2/1
  Subtract1/1 -> Subtract2/2, Scope/1
  Subtract2/1 -> Out1/1
  Step3/1 -> Subtract1/2

== system ARC_DTm/Plant_LocalLoad_FMU/Battery System/Battery PID Solar Data3/open-loop steps ==
  Scope : Scope
      settings: ActiveDisplayYMinimum=-1.125  ActiveDisplayYMaximum=0.125
  Step : Step  Time=10000  SampleTime=0
  Step1 : Step  Time=46500  After=-1  SampleTime=0
  Step2 : Step  Time=60000  After=-1  SampleTime=0
  Step3 : Step  Time=90000  SampleTime=0
  Subtract : Sum
  Subtract1 : Sum
  Subtract2 : Sum
  Out1 : Outport
  wires:
  Step/1 -> Subtract/1
  Step1/1 -> Subtract/2
  Step2/1 -> Subtract1/1
  Subtract/1 -> Subtract2/1
  Subtract1/1 -> Subtract2/2, Scope/1
  Subtract2/1 -> Out1/1
  Step3/1 -> Subtract1/2

== system ARC_DTm/Plant_LocalLoad_FMU/Battery System/Excess Solar/Battery PID Solar Data ==
  note: M=2.5, kp=2.965, Ti=166.5, ki=0.0178
      |
      | M=1.5, kp=4.9, Ti=99.9, ki=0.049
      |
      | M=0.5, kp=14.8, Ti=33.3, ki=0.4
      |
      | M=0.1, kp=74.13, Ti=6.66, ki=11.13
      |
      | M=0.055 kp=134.79, Ti=3.663, ki=36.79
      |
      | M=0.01, kp=741.35, Ti=0.666, ki=1112.8
      |
      | M=0.001, kp=7413.5, Ti=0.0666, ki=111,313.81
      |
      | M=0.0001, kp=74135.09, Ti=0.00666, ki=11,113,394.89
  Setpoint : Inport
  feedback : Inport  Port=2
  Add : Sum
  BatteryCharge : Saturate  UpperLimit=1  LowerLimit=0
  Constant : Constant  Value=0
  Dead Zone : DeadZone  LowerValue=-0.01  UpperValue=0.01
  Dead Zone1 : DeadZone  LowerValue=-0.025  UpperValue=0.025
  Gain7 : Gain  Gain=134.79
  Gain8 : Gain  Gain=36.79
  Manual Switch : ManualSwitch
  Proportional3 : Gain  SaturateOnIntegerOverflow=on  OutDataTypeStr=Inherit: Same as input  ParamDataTypeStr=Inherit: Same as input
  Scope : Scope  NumInputPorts=3
      settings: ActiveDisplayYMinimum=-119.32425521603426  ActiveDisplayYMaximum=13.258250579559359  DataLoggingVariableName=ScopeData4
  Scope1 : Scope
      settings: ActiveDisplayYMinimum=-1  ActiveDisplayYMaximum=1  DataLoggingVariableName=ScopeData9
  Scope2 : Scope  NumInputPorts=4
      settings: Title=Setpoint  ActiveDisplayYMinimum=-0.96522618502196855  ActiveDisplayYMaximum=1.0322332055334107  DataLoggingVariableName=ScopeData2
  Scope3 : Scope  NumInputPorts=2
      settings: ActiveDisplayYMinimum=-0.25471317003362626  ActiveDisplayYMaximum=0.79251853030263664  DataLoggingVariableName=ScopeData2
  Subtract : Sum  Inputs=+-
  Subtract1 : Sum  Inputs=+-
  Sum1 : Sum  Inputs=|+-
  Sum6 : Sum  Inputs=+-  InputSameDT=on  SaturateOnIntegerOverflow=on  OutDataTypeStr=Inherit: Same as first input
  Unit Delay : UnitDelay  SampleTime=-1  HasFrameUpgradeWarning=on
  open-loop steps : Subsystem
  BatteryChargeDisch : Outport
  wires:
  Manual Switch/1 -> BatteryChargeDisch/1
  open-loop steps/1(Out1) -> Manual Switch/2
  Setpoint/1 -> Scope2/1, Subtract1/1
  Proportional3/1 -> Subtract/2
  feedback/1 -> Scope2/2, Subtract1/2
  Sum1/1 -> Add/2, Unit Delay/1
  Subtract/1 -> Scope1/1, Sum1/1
  Unit Delay/1 -> Sum1/2
  Subtract1/1 -> Scope3/2, Gain8/1, Gain7/1, Scope2/3, Scope3/1
  BatteryCharge/1 -> Scope2/4, Manual Switch/1, Sum6/2, Scope/2
  Add/1 -> Scope/1, Sum6/1, BatteryCharge/1
  Gain7/1 -> Add/1
  Gain8/1 -> Subtract/1
  Sum6/1 -> Proportional3/1, Scope/3

== system ARC_DTm/Plant_LocalLoad_FMU/Battery System/Excess Solar/Battery PID Solar Data1 ==
  note: M=2.5, kp=2.965, Ti=166.5, ki=0.0178
      |
      | M=1.5, kp=4.9, Ti=99.9, ki=0.049
      |
      | M=0.5, kp=14.8, Ti=33.3, ki=0.4
      |
      | M=0.1, kp=74.13, Ti=6.66, ki=11.13
      |
      | M=0.055 kp=134.79, Ti=3.663, ki=36.79
      |
      | M=0.01, kp=741.35, Ti=0.666, ki=1112.8
      |
      | M=0.001, kp=7413.5, Ti=0.0666, ki=111,313.81
      |
      | M=0.0001, kp=74135.09, Ti=0.00666, ki=11,113,394.89
  Setpoint : Inport
  feedback : Inport  Port=2
  Add : Sum
  BatteryCharge : Saturate  UpperLimit=0  LowerLimit=-1
  Constant : Constant  Value=0
  Dead Zone : DeadZone  LowerValue=-0.01  UpperValue=0.01
  Dead Zone1 : DeadZone  LowerValue=-0.025  UpperValue=0.025
  Gain7 : Gain  Gain=134.79
  Gain8 : Gain  Gain=36.79
  Manual Switch : ManualSwitch
  Proportional3 : Gain  SaturateOnIntegerOverflow=on  OutDataTypeStr=Inherit: Same as input  ParamDataTypeStr=Inherit: Same as input
  Scope : Scope  NumInputPorts=3
      settings: ActiveDisplayYMinimum=-113.50359317586926  ActiveDisplayYMaximum=90.190900765776917  DataLoggingVariableName=ScopeData4
  Scope1 : Scope
      settings: ActiveDisplayYMinimum=-1  ActiveDisplayYMaximum=1  DataLoggingVariableName=ScopeData8
  Scope2 : Scope  NumInputPorts=4
      settings: Title=Setpoint  ActiveDisplayYMinimum=-0.96522618550308326  ActiveDisplayYMaximum=1.0322332098634432  DataLoggingVariableName=ScopeData2
  Subtract : Sum  Inputs=+-
  Subtract1 : Sum  Inputs=+-
  Sum1 : Sum  Inputs=|+-
  Sum6 : Sum  Inputs=+-  InputSameDT=on  SaturateOnIntegerOverflow=on  OutDataTypeStr=Inherit: Same as first input
  Unit Delay : UnitDelay  SampleTime=-1  HasFrameUpgradeWarning=on
  Unit Delay1 : UnitDelay  SampleTime=-1  HasFrameUpgradeWarning=on
  open-loop steps : Subsystem
  Battery Disch : Outport
  wires:
  Manual Switch/1 -> Battery Disch/1
  open-loop steps/1(Out1) -> Manual Switch/2
  Setpoint/1 -> Scope2/1, Subtract1/1
  Proportional3/1 -> Subtract/2
  feedback/1 -> Scope2/2, Subtract1/2
  Sum1/1 -> Add/2, Unit Delay/1
  Subtract/1 -> Scope1/1, Sum1/1
  Unit Delay/1 -> Sum1/2
  Subtract1/1 -> Gain8/1, Gain7/1, Scope2/3
  BatteryCharge/1 -> Sum6/2, Scope2/4, Manual Switch/1, Scope/2
  Add/1 -> Scope/1, BatteryCharge/1, Sum6/1
  Gain7/1 -> Add/1
  Gain8/1 -> Subtract/1
  Sum6/1 -> Proportional3/1, Scope/3

== system ARC_DTm/Plant_LocalLoad_FMU/Battery System/Excess Solar/Setpoint PID Solar+Battery  ==
  Solar Power : Inport
  Local Load Demand : Inport  Port=2
  Divide : Product  Inputs=*/
  Rate Limiter1 : RateLimiter  RisingSlewLimit=0.00000607  FallingSlewLimit=-0.00000607  SampleTimeMode=inherited
  Rate Limiter2 : RateLimiter  RisingSlewLimit=0.00000607  FallingSlewLimit=-0.00000607  SampleTimeMode=inherited
  Saturation1 : Saturate  UpperLimit=0.9  LowerLimit=-0.9
  Saturation4 : Saturate  UpperLimit=0.9  LowerLimit=-0.9
  Scaling factor Solar Data to 1 MW Battery : Constant  Value=10000
  Scope7 : Scope  NumInputPorts=3
      settings: Title=Battery Charge/Discharge SOC Output  ActiveDisplayYMinimum=-0.95011803109224124  ActiveDisplayYMaximum=0.10556867012136011
  Subtract2 : Sum  Inputs=+-
  Transfer Fcn3 : TransferFcn  Denominator=[300 1]
  Setpoint BattCharge : Outport
  Setpoint BattDischarge : Outport  Port=2
  wires:
  Subtract2/1 -> Scope7/1, Transfer Fcn3/1
  Transfer Fcn3/1 -> Divide/1
  Local Load Demand/1 -> Subtract2/2
  Solar Power/1 -> Subtract2/1
  Divide/1 -> Saturation1/1, Saturation4/1
  Saturation4/1 -> Setpoint BattCharge/1, Scope7/2
  Saturation1/1 -> Scope7/3, Setpoint BattDischarge/1
  Scaling factor Solar Data to 1 MW Battery/1 -> Divide/2

== system ARC_DTm/Product Water Tank/Tank Storage/Manage Overflows/If Action Subsystem ==
  <Flow Rate (FLOW)> : Inport
  <Permeate Flow (FLOW)> : Inport  Port=2
  Pump Flow (FLOW) : Inport  Port=3
  Action Port : ActionPort
  Gain : Gain  Gain=.95
  Normalized RO Perm Inflow : Product
  Normalized Well Inflow : Product
  Percent RO Perm Inflow : Product  Inputs=/*
  Percent Well Inflow : Product  Inputs=*/
  Total Inflow : Sum  Inputs=|++
  Raw Water Flow Rate (FLOW) : Outport
  RO Permeate Flow Rate (FLOW) : Outport  Port=2
  Pump Flow Rate (FLOW) : Outport  Port=3
  wires:
  <Flow Rate (FLOW)>/1 -> Percent Well Inflow/1, Total Inflow/1
  <Permeate Flow (FLOW)>/1 -> Percent RO Perm Inflow/2, Total Inflow/2
  Total Inflow/1 -> Percent RO Perm Inflow/1, Percent Well Inflow/2
  Percent Well Inflow/1 -> Normalized Well Inflow/1
  Pump Flow (FLOW)/1 -> Pump Flow Rate (FLOW)/1, Gain/1
  Percent RO Perm Inflow/1 -> Normalized RO Perm Inflow/1
  Normalized Well Inflow/1 -> Raw Water Flow Rate (FLOW)/1  "Well Inflow (FLOW)"
  Normalized RO Perm Inflow/1 -> RO Permeate Flow Rate (FLOW)/1  "RO Permeate Inflow (FLOW)"
  Gain/1 -> Normalized RO Perm Inflow/2, Normalized Well Inflow/2

== system ARC_DTm/Product Water Tank/Tank Storage/Manage Overflows/If Action Subsystem1 ==
  <Flow Rate (FLOW)> : Inport
  <Permeate Flow (FLOW)> : Inport  Port=2
  <Pump Flow (FLOW)> : Inport  Port=3
  Action Port : ActionPort
  Well Flow Rate (FLOW) : Outport
  RO Perm Flow Rate (FLOW) : Outport  Port=2
  Pump Flow (FLOW) : Outport  Port=3
  wires:
  <Flow Rate (FLOW)>/1 -> Well Flow Rate (FLOW)/1
  <Permeate Flow (FLOW)>/1 -> RO Perm Flow Rate (FLOW)/1
  <Pump Flow (FLOW)>/1 -> Pump Flow (FLOW)/1

== system ARC_DTm/Product Water Tank/Tank Storage/Manage Overflows/Pump Flow Reduction ==
  <Flow Rate (FLOW)> : Inport
  <PermeateFlow (FLOW)> : Inport  Port=2
  Action Port : ActionPort
  Gain : Gain  Gain=.95
  Sum : Sum  Inputs=|++
  Well Flow Rate (FLOW) : Outport
  Permeate Flow Rate (FLOW) : Outport  Port=2
  Pump Flow (FLOW) : Outport  Port=3
  wires:
  <Flow Rate (FLOW)>/1 -> Well Flow Rate (FLOW)/1, Sum/1
  <PermeateFlow (FLOW)>/1 -> Permeate Flow Rate (FLOW)/1, Sum/2
  Sum/1 -> Gain/1  "Pump Flow (FLOW)"
  Gain/1 -> Pump Flow (FLOW)/1

== system ARC_DTm/Product Water Tank/Tank Storage/VolumeConditions/Tank Above Operating Range ==
  Action Port : ActionPort
  Tank Overflow? : Constant  Value=15
  Out1 : Outport
  wires:
  Tank Overflow?/1 -> Out1/1

== system ARC_DTm/Product Water Tank/Tank Storage/VolumeConditions/Tank Below Operating Range ==
  Action Port : ActionPort
  Tank Empty : Constant  Value=-15
  Out1 : Outport
  wires:
  Tank Empty/1 -> Out1/1

== system ARC_DTm/Product Water Tank/Tank Storage/VolumeConditions/Tank in Operating Range ==
  Timer : Inport
  Action Port : ActionPort
  y : Outport
  wires:
  ? -> y/1

== system ARC_DTm/Plant_LocalLoad_FMU/Battery System/Excess Solar/Battery PID Solar Data/open-loop steps ==
  Scope : Scope
      settings: ActiveDisplayYMinimum=-1.125  ActiveDisplayYMaximum=0.125
  Step : Step  Time=10000  SampleTime=0
  Step1 : Step  Time=46500  After=-1  SampleTime=0
  Step2 : Step  Time=60000  After=-1  SampleTime=0
  Step3 : Step  Time=90000  SampleTime=0
  Subtract : Sum
  Subtract1 : Sum
  Subtract2 : Sum
  Out1 : Outport
  wires:
  Step/1 -> Subtract/1
  Step1/1 -> Subtract/2
  Step2/1 -> Subtract1/1
  Subtract/1 -> Subtract2/1
  Subtract1/1 -> Subtract2/2, Scope/1
  Subtract2/1 -> Out1/1
  Step3/1 -> Subtract1/2

== system ARC_DTm/Plant_LocalLoad_FMU/Battery System/Excess Solar/Battery PID Solar Data1/open-loop steps ==
  Scope : Scope
      settings: ActiveDisplayYMinimum=-1.125  ActiveDisplayYMaximum=0.125
  Step : Step  Time=10000  SampleTime=0
  Step1 : Step  Time=46500  After=-1  SampleTime=0
  Step2 : Step  Time=60000  After=-1  SampleTime=0
  Step3 : Step  Time=90000  SampleTime=0
  Subtract : Sum
  Subtract1 : Sum
  Subtract2 : Sum
  Out1 : Outport
  wires:
  Step/1 -> Subtract/1
  Step1/1 -> Subtract/2
  Step2/1 -> Subtract1/1
  Subtract/1 -> Subtract2/1
  Subtract1/1 -> Subtract2/2, Scope/1
  Subtract2/1 -> Out1/1
  Step3/1 -> Subtract1/2
